simulink model "PMSM20180521"  (Simulink 7.9)
settings: Solver=FixedStepDiscrete  StartTime=0.0  StopTime=1  FixedStep=Auto  RelTol=1e-3
undefined symbols (not defined in the file or in its folder): Down, Up
libraries: idelinklib_common x37, simulink x13, c2833xlib x7, c280xlib x6, simulink_extras x2, idelinklib_ticcs x1, idelinklib_tgtpref x1
(part 2 of 3)

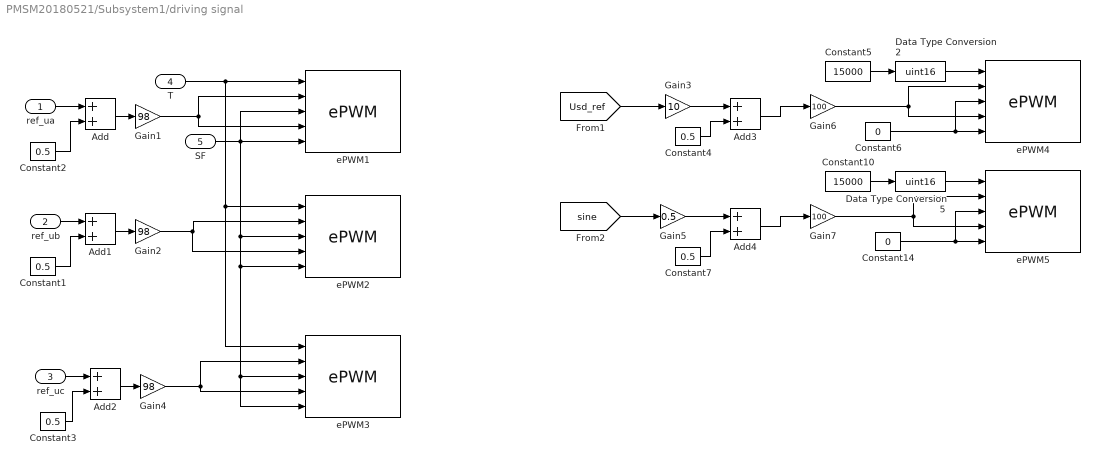
== system PMSM20180521/Subsystem1/driving signal ==
  ref_ua : Inport
  ref_ub : Inport  Port=2
  ref_uc : Inport  Port=3
  T : Inport  Port=4
  SF : Inport  Port=5
  Add{,1..4} (5 alike) : Sum
  Constant{1..4,7} (5 alike) : Constant  Value=0.5  OutDataTypeStr=double
  Constant10 : Constant  Value=15000  OutDataTypeStr=int16
  Constant14 : Constant  Value=0  OutDataTypeStr=boolean
  Constant5 : Constant  Value=15000  OutDataTypeStr=int16
  Constant6 : Constant  Value=0  OutDataTypeStr=boolean
  Data Type Conversion2 : DataTypeConversion  OutDataTypeStr=uint16
  Data Type Conversion5 : DataTypeConversion  OutDataTypeStr=uint16
  Gain1 : Gain  Gain=98
  Gain2 : Gain  Gain=98
  Gain3 : Gain  Gain=10
  Gain4 : Gain  Gain=98
  Gain5 : Gain  Gain=0.5
  Gain6 : Gain  Gain=100
  Gain7 : Gain  Gain=100
  ePWM1 : c280xlib/ePWM  checkMode=off  useModule=ePWM1  periodUnits=Clock cycles  timerSource=Input port  timerPeriod_clk=15000  timerPeriod_sec=1/20000  countingMode=Up-Down  synchronizationOption=CTR=Zero  synchronizationEnable=off  phaseActiveEnable=Disable  phaseDirection=Count down after sync  phaseActive=0  clockPrescale=1  HSclockPrescale=1  ePWMxAStatus=off  CMPAUnits=Percentages  CMPASource=Input port  CMPAValue_per=0  CMPAValue_clk=32000  ePWMxAactionLogic1=Do nothing  ePWMxAactionLogic2=Do nothing  ePWMxAactionLogic3=Clear  ePWMxAactionLogic4=Set  ePWMxAactionLogic5=Do nothing  ePWMxAactionLogic6=Do nothing  ePWMxALoadMode=Load on CTR=Zero  ePWMxACSFenable=on  ePWMxACSFvalue=Forcing Disable  ePWMxASFreload=Zero  enHRPWM=off  HRPWM_LoadMode=CTR=ZERO  HRPWM_CTLMode=Phase control mode  HRPWM_EDGMode=Both edge  enSFO=on  ePWMxBStatus=on  CMPBUnits=Percentages  CMPBSource=Input port  CMPBValue_per=0  CMPBValue_clk=32000  ePWMxBactionLogic1=Do nothing  ePWMxBactionLogic2=Do nothing  ePWMxBactionLogic3=Do nothing  ePWMxBactionLogic4=Do nothing  ePWMxBactionLogic5=Set  ePWMxBactionLogic6=Clear  ePWMxBLoadMode=Load on CTR=Zero  ePWMxBCSFenable=on  ePWMxBCSFvalue=Forcing Disable  ePWMxBSFreload=Zero  enableDBePWMxA=on  enableDBePWMxB=on  DBpolarity=AHC  DBedgeDelay=Positive  DBSource_ePWMxA=ePWMxB  DBSource_ePWMxB=ePWMxB  DBperiodSource=Specify via dialog  REDperiod=525  FEDperiod=525  adcstartModuleA=off  adcrequestEventA=First event  adcstartEventA=CTR=Zero  adcstartModuleB=off  adcrequestEventB=First event  adcstartEventB=CTR=Zero  intEn=on  intPrd=First event  intSel=CTR=Zero  chopperEnable=off  chopperFrequency=1  chopperFirstwidth=1  chopperDuty=12.5%  tripZonesource=Specify via dialog  tzselOSHT1=off  tzselOSHT2=off  tzselOSHT3=off  tzselOSHT4=off  tzselOSHT5=off  tzselOSHT6=off  tzselCBC1=off  tzselCBC2=off  tzselCBC3=off  tzselCBC4=off  tzselCBC5=off  tzselCBC6=off  enTzOstIntr=off  enTzCbcIntr=off  ePWMxAforced=No action  ePWMxBforced=No action  timerPeriod=-1  ePWMxAValue=0  ePWMxBValue=0  tripZoneoption=OSHT
  ePWM2 : c280xlib/ePWM  checkMode=off  useModule=ePWM2  periodUnits=Clock cycles  timerSource=Input port  timerPeriod_clk=15000  timerPeriod_sec=1/20000  countingMode=Up-Down  synchronizationOption=EPWMxSYNCI or SWFSYNC  synchronizationEnable=off  phaseActiveEnable=Specify via dialog  phaseDirection=Count up after sync  phaseActive=0  clockPrescale=1  HSclockPrescale=1  ePWMxAStatus=off  CMPAUnits=Percentages  CMPASource=Input port  CMPAValue_per=0  CMPAValue_clk=32000  ePWMxAactionLogic1=Do nothing  ePWMxAactionLogic2=Do nothing  ePWMxAactionLogic3=Clear  ePWMxAactionLogic4=Set  ePWMxAactionLogic5=Do nothing  ePWMxAactionLogic6=Do nothing  ePWMxALoadMode=Load on CTR=Zero  ePWMxACSFenable=on  ePWMxACSFvalue=Forcing Disable  ePWMxASFreload=Zero  enHRPWM=off  HRPWM_LoadMode=CTR=ZERO  HRPWM_CTLMode=Phase control mode  HRPWM_EDGMode=Both edge  enSFO=on  ePWMxBStatus=on  CMPBUnits=Percentages  CMPBSource=Input port  CMPBValue_per=0  CMPBValue_clk=32000  ePWMxBactionLogic1=Do nothing  ePWMxBactionLogic2=Do nothing  ePWMxBactionLogic3=Do nothing  ePWMxBactionLogic4=Do nothing  ePWMxBactionLogic5=Set  ePWMxBactionLogic6=Clear  ePWMxBLoadMode=Load on CTR=Zero  ePWMxBCSFenable=on  ePWMxBCSFvalue=Forcing Disable  ePWMxBSFreload=Zero  enableDBePWMxA=on  enableDBePWMxB=on  DBpolarity=AHC  DBedgeDelay=Positive  DBSource_ePWMxA=ePWMxB  DBSource_ePWMxB=ePWMxB  DBperiodSource=Specify via dialog  REDperiod=525  FEDperiod=525  adcstartModuleA=off  adcrequestEventA=First event  adcstartEventA=CTR=Zero  adcstartModuleB=off  adcrequestEventB=First event  adcstartEventB=CTR=Zero  intEn=off  intPrd=First event  intSel=CTR=Zero  chopperEnable=off  chopperFrequency=1  chopperFirstwidth=1  chopperDuty=12.5%  tripZonesource=Specify via dialog  tzselOSHT1=off  tzselOSHT2=off  tzselOSHT3=off  tzselOSHT4=off  tzselOSHT5=off  tzselOSHT6=off  tzselCBC1=off  tzselCBC2=off  tzselCBC3=off  tzselCBC4=off  tzselCBC5=off  tzselCBC6=off  enTzOstIntr=off  enTzCbcIntr=off  ePWMxAforced=No action  ePWMxBforced=No action  timerPeriod=-1  ePWMxAValue=0  ePWMxBValue=0  tripZoneoption=OSHT
  ePWM3 : c280xlib/ePWM  checkMode=off  useModule=ePWM3  periodUnits=Clock cycles  timerSource=Input port  timerPeriod_clk=15000  timerPeriod_sec=1/20000  countingMode=Up-Down  synchronizationOption=EPWMxSYNCI or SWFSYNC  synchronizationEnable=off  phaseActiveEnable=Specify via dialog  phaseDirection=Count up after sync  phaseActive=0  clockPrescale=1  HSclockPrescale=1  ePWMxAStatus=off  CMPAUnits=Percentages  CMPASource=Input port  CMPAValue_per=0  CMPAValue_clk=32000  ePWMxAactionLogic1=Do nothing  ePWMxAactionLogic2=Do nothing  ePWMxAactionLogic3=Clear  ePWMxAactionLogic4=Set  ePWMxAactionLogic5=Do nothing  ePWMxAactionLogic6=Do nothing  ePWMxALoadMode=Load on CTR=Zero  ePWMxACSFenable=on  ePWMxACSFvalue=Forcing Disable  ePWMxASFreload=Zero  enHRPWM=off  HRPWM_LoadMode=CTR=ZERO  HRPWM_CTLMode=Phase control mode  HRPWM_EDGMode=Both edge  enSFO=on  ePWMxBStatus=on  CMPBUnits=Percentages  CMPBSource=Input port  CMPBValue_per=0  CMPBValue_clk=32000  ePWMxBactionLogic1=Do nothing  ePWMxBactionLogic2=Do nothing  ePWMxBactionLogic3=Do nothing  ePWMxBactionLogic4=Do nothing  ePWMxBactionLogic5=Set  ePWMxBactionLogic6=Clear  ePWMxBLoadMode=Load on CTR=Zero  ePWMxBCSFenable=on  ePWMxBCSFvalue=Forcing Disable  ePWMxBSFreload=Zero  enableDBePWMxA=on  enableDBePWMxB=on  DBpolarity=AHC  DBedgeDelay=Positive  DBSource_ePWMxA=ePWMxB  DBSource_ePWMxB=ePWMxB  DBperiodSource=Specify via dialog  REDperiod=525  FEDperiod=525  adcstartModuleA=off  adcrequestEventA=First event  adcstartEventA=CTR=Zero  adcstartModuleB=off  adcrequestEventB=First event  adcstartEventB=CTR=Zero  intEn=off  intPrd=First event  intSel=CTR=Zero  chopperEnable=off  chopperFrequency=1  chopperFirstwidth=1  chopperDuty=12.5%  tripZonesource=Specify via dialog  tzselOSHT1=off  tzselOSHT2=off  tzselOSHT3=off  tzselOSHT4=off  tzselOSHT5=off  tzselOSHT6=off  tzselCBC1=off  tzselCBC2=off  tzselCBC3=off  tzselCBC4=off  tzselCBC5=off  tzselCBC6=off  enTzOstIntr=off  enTzCbcIntr=off  ePWMxAforced=No action  ePWMxBforced=No action  timerPeriod=-1  ePWMxAValue=0  ePWMxBValue=0  tripZoneoption=OSHT
  ePWM4 : c280xlib/ePWM  checkMode=off  useModule=ePWM4  periodUnits=Clock cycles  timerSource=Input port  timerPeriod_clk=15000  timerPeriod_sec=1/20000  countingMode=Up-Down  synchronizationOption=EPWMxSYNCI or SWFSYNC  synchronizationEnable=off  phaseActiveEnable=Specify via dialog  phaseDirection=Count up after sync  phaseActive=0  clockPrescale=1  HSclockPrescale=1  ePWMxAStatus=on  CMPAUnits=Percentages  CMPASource=Input port  CMPAValue_per=0  CMPAValue_clk=32000  ePWMxAactionLogic1=Do nothing  ePWMxAactionLogic2=Do nothing  ePWMxAactionLogic3=Clear  ePWMxAactionLogic4=Set  ePWMxAactionLogic5=Do nothing  ePWMxAactionLogic6=Do nothing  ePWMxALoadMode=Load on CTR=Zero  ePWMxACSFenable=on  ePWMxACSFvalue=Forcing Disable  ePWMxASFreload=Zero  enHRPWM=off  HRPWM_LoadMode=CTR=ZERO  HRPWM_CTLMode=Phase control mode  HRPWM_EDGMode=Both edge  enSFO=on  ePWMxBStatus=on  CMPBUnits=Percentages  CMPBSource=Input port  CMPBValue_per=0  CMPBValue_clk=32000  ePWMxBactionLogic1=Do nothing  ePWMxBactionLogic2=Do nothing  ePWMxBactionLogic3=Do nothing  ePWMxBactionLogic4=Do nothing  ePWMxBactionLogic5=Clear  ePWMxBactionLogic6=Set  ePWMxBLoadMode=Load on CTR=Zero  ePWMxBCSFenable=on  ePWMxBCSFvalue=Forcing Disable  ePWMxBSFreload=Zero  enableDBePWMxA=off  enableDBePWMxB=off  DBpolarity=AHC  DBedgeDelay=Positive  DBSource_ePWMxA=ePWMxB  DBSource_ePWMxB=ePWMxB  DBperiodSource=Specify via dialog  REDperiod=0  FEDperiod=0  adcstartModuleA=off  adcrequestEventA=First event  adcstartEventA=CTR=Zero  adcstartModuleB=off  adcrequestEventB=First event  adcstartEventB=CTR=Zero  intEn=off  intPrd=First event  intSel=CTR=Zero  chopperEnable=off  chopperFrequency=1  chopperFirstwidth=1  chopperDuty=12.5%  tripZonesource=Specify via dialog  tzselOSHT1=off  tzselOSHT2=off  tzselOSHT3=off  tzselOSHT4=off  tzselOSHT5=off  tzselOSHT6=off  tzselCBC1=off  tzselCBC2=off  tzselCBC3=off  tzselCBC4=off  tzselCBC5=off  tzselCBC6=off  enTzOstIntr=off  enTzCbcIntr=off  ePWMxAforced=No action  ePWMxBforced=No action  timerPeriod=-1  ePWMxAValue=0  ePWMxBValue=0  tripZoneoption=OSHT
  ePWM5 : c280xlib/ePWM  checkMode=off  useModule=ePWM5  periodUnits=Clock cycles  timerSource=Input port  timerPeriod_clk=15000  timerPeriod_sec=1/20000  countingMode=Up-Down  synchronizationOption=EPWMxSYNCI or SWFSYNC  synchronizationEnable=off  phaseActiveEnable=Specify via dialog  phaseDirection=Count up after sync  phaseActive=0  clockPrescale=1  HSclockPrescale=1  ePWMxAStatus=on  CMPAUnits=Percentages  CMPASource=Input port  CMPAValue_per=0  CMPAValue_clk=32000  ePWMxAactionLogic1=Do nothing  ePWMxAactionLogic2=Do nothing  ePWMxAactionLogic3=Clear  ePWMxAactionLogic4=Set  ePWMxAactionLogic5=Do nothing  ePWMxAactionLogic6=Do nothing  ePWMxALoadMode=Load on CTR=Zero  ePWMxACSFenable=on  ePWMxACSFvalue=Forcing Disable  ePWMxASFreload=Zero  enHRPWM=off  HRPWM_LoadMode=CTR=ZERO  HRPWM_CTLMode=Phase control mode  HRPWM_EDGMode=Both edge  enSFO=on  ePWMxBStatus=on  CMPBUnits=Percentages  CMPBSource=Input port  CMPBValue_per=0  CMPBValue_clk=32000  ePWMxBactionLogic1=Do nothing  ePWMxBactionLogic2=Do nothing  ePWMxBactionLogic3=Do nothing  ePWMxBactionLogic4=Do nothing  ePWMxBactionLogic5=Clear  ePWMxBactionLogic6=Set  ePWMxBLoadMode=Load on CTR=Zero  ePWMxBCSFenable=on  ePWMxBCSFvalue=Forcing Disable  ePWMxBSFreload=Zero  enableDBePWMxA=off  enableDBePWMxB=off  DBpolarity=AHC  DBedgeDelay=Positive  DBSource_ePWMxA=ePWMxB  DBSource_ePWMxB=ePWMxB  DBperiodSource=Specify via dialog  REDperiod=0  FEDperiod=0  adcstartModuleA=off  adcrequestEventA=First event  adcstartEventA=CTR=Zero  adcstartModuleB=off  adcrequestEventB=First event  adcstartEventB=CTR=Zero  intEn=off  intPrd=First event  intSel=CTR=Zero  chopperEnable=off  chopperFrequency=1  chopperFirstwidth=1  chopperDuty=12.5%  tripZonesource=Specify via dialog  tzselOSHT1=off  tzselOSHT2=off  tzselOSHT3=off  tzselOSHT4=off  tzselOSHT5=off  tzselOSHT6=off  tzselCBC1=off  tzselCBC2=off  tzselCBC3=off  tzselCBC4=off  tzselCBC5=off  tzselCBC6=off  enTzOstIntr=off  enTzCbcIntr=off  ePWMxAforced=No action  ePWMxBforced=No action  timerPeriod=-1  ePWMxAValue=0  ePWMxBValue=0  tripZoneoption=OSHT
  wires:
  SF/1 -> ePWM1/3, ePWM1/5, ePWM3/5, ePWM3/3, ePWM2/5, ePWM2/3
  T/1 -> ePWM1/1, ePWM3/1, ePWM2/1
  ref_ua/1 -> Add/1
  Add/1 -> Gain1/1
  Constant2/1 -> Add/2
  Gain1/1 -> ePWM1/2, ePWM1/4
  ref_ub/1 -> Add1/1
  Constant1/1 -> Add1/2
  Add1/1 -> Gain2/1
  Gain2/1 -> ePWM2/4, ePWM2/2
  ref_uc/1 -> Add2/1
  Constant3/1 -> Add2/2
  Add2/1 -> Gain4/1
  Gain4/1 -> ePWM3/2, ePWM3/4
  Data Type Conversion5/1 -> ePWM5/1
  Constant14/1 -> ePWM5/3, ePWM5/5
  Constant5/1 -> Data Type Conversion2/1
  Gain7/1 -> ePWM5/2, ePWM5/4
  Data Type Conversion2/1 -> ePWM4/1
  Gain6/1 -> ePWM4/4, ePWM4/2
  Constant10/1 -> Data Type Conversion5/1
  Constant6/1 -> ePWM4/3, ePWM4/5
  [sine] -> Gain5/1
  [Usd_ref] -> Gain3/1
  Gain3/1 -> Add3/1
  Add3/1 -> Gain6/1
  Constant4/1 -> Add3/2
  Gain5/1 -> Add4/1
  Add4/1 -> Gain7/1
  Constant7/1 -> Add4/2

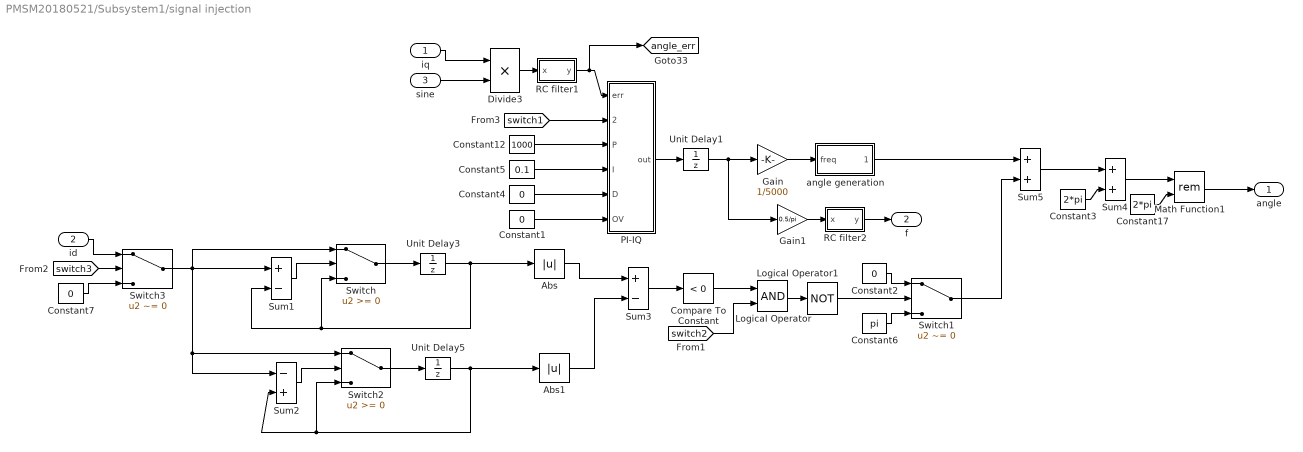
== system PMSM20180521/Subsystem1/signal injection ==
  iq : Inport
  id : Inport  Port=2
  sine : Inport  Port=3
  Abs : Abs
  Abs1 : Abs
  Compare To Constant : simulink/Logic and Bit Operations/Compare To Constant  relop=<  const=0  OutDataTypeStr=boolean
  Constant{1..2,4,7} (4 alike) : Constant  Value=0  OutDataTypeStr=double
  Constant12 : Constant  Value=1000  OutDataTypeStr=double
  Constant17 : Constant  Value=2*pi  OutDataTypeStr=double
  Constant3 : Constant  Value=2*pi  OutDataTypeStr=double
  Constant5 : Constant  Value=0.1  OutDataTypeStr=double
  Constant6 : Constant  Value=pi  OutDataTypeStr=double
  Divide3 : Product  Inputs=**
  Gain : Gain  Gain=1/5000
  Gain1 : Gain  Gain=0.5/pi
  Logical Operator : Logic  AllPortsSameDT=off  OutDataTypeStr=boolean
  Logical Operator1 : Logic  Operator=NOT  AllPortsSameDT=off  OutDataTypeStr=boolean
  Math Function1 : Math  Operator=rem  SaturateOnIntegerOverflow=on
  PI-IQ : Subsystem  mask{ermax=100, ermin=-100, max=300, min=-300}
      mask prompts: ermax "Err max limit"; ermin "Err min limit"; max "Output max limit"; min "Output min limit"
  RC filter1 : Subsystem  mask{a=0.05}
      mask prompts: a "Time Constant"
  RC filter2 : Subsystem  mask{a=0.05}
      mask prompts: a "Time Constant"
  Sum1 : Sum  Inputs=+-
  Sum2 : Sum  Inputs=-+
  Sum3 : Sum  Inputs=+-
  Sum4 : Sum
  Sum5 : Sum
  Switch : Switch
  Switch1 : Switch  Criteria=u2 ~= 0
  Switch2 : Switch
  Switch3 : Switch  Criteria=u2 ~= 0
  Unit Delay1 : UnitDelay  SampleTime=-1
  Unit Delay3 : UnitDelay  SampleTime=-1
  Unit Delay5 : UnitDelay  SampleTime=-1
  angle generation : Subsystem
  angle : Outport
  f : Outport  Port=2
  tag scope: angle_err=global
  wires:
  sine/1 -> Divide3/2
  Divide3/1 -> RC filter1/1(x)
  Constant12/1 -> PI-IQ/3(P)
  Constant5/1 -> PI-IQ/4(I)
  Constant4/1 -> PI-IQ/5(D)
  Constant1/1 -> PI-IQ/6(OV)
  RC filter1/1(y) -> PI-IQ/1(err), [angle_err]
  PI-IQ/1(out) -> Unit Delay1/1
  iq/1 -> Divide3/1
  Gain/1 -> angle generation/1(freq)
  Unit Delay1/1 -> Gain/1, Gain1/1
  Gain1/1 -> RC filter2/1(x)
  Constant3/1 -> Sum4/2
  Constant17/1 -> Math Function1/2
  Sum4/1 -> Math Function1/1
  Math Function1/1 -> angle/1
  RC filter2/1(y) -> f/1
  [switch1] -> PI-IQ/2(reset)
  Sum1/1 -> Switch/2
  Switch/1 -> Unit Delay3/1
  Unit Delay3/1 -> Sum1/2, Switch/3, Abs/1
  Sum2/1 -> Switch2/2
  Switch2/1 -> Unit Delay5/1
  Unit Delay5/1 -> Sum2/2, Switch2/3, Abs1/1
  Abs/1 -> Sum3/1
  Abs1/1 -> Sum3/2
  Constant2/1 -> Switch1/1
  Constant6/1 -> Switch1/3
  Sum3/1 -> Compare To Constant/1
  Compare To Constant/1 -> Logical Operator/1
  [switch2] -> Logical Operator/2
  Logical Operator/1 -> Logical Operator1/1
  Logical Operator1/1 -> Switch1/2
  Switch3/1 -> Sum1/1, Switch/1, Sum2/1, Switch2/1
  [switch3] -> Switch3/2
  id/1 -> Switch3/1
  Constant7/1 -> Switch3/3
  Sum5/1 -> Sum4/1
  Switch1/1 -> Sum5/2
  angle generation/1(angle_0) -> Sum5/1

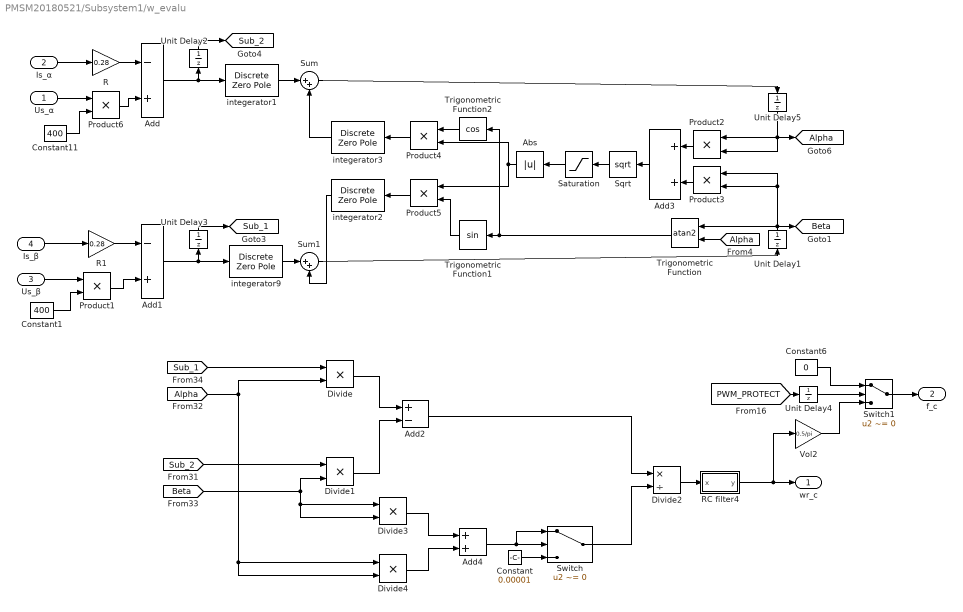
== system PMSM20180521/Subsystem1/w_evalu ==
  Us_α : Inport
  Is_α : Inport  Port=2
  Us_β : Inport  Port=3
  Is_β : Inport  Port=4
  Abs : Abs
  Add : Sum  Inputs=-+
  Add1 : Sum  Inputs=-+
  Add2 : Sum  Inputs=+-
  Add3 : Sum
  Add4 : Sum
  Constant : Constant  Value=0.00001
  Constant1 : Constant  Value=400  OutDataTypeStr=double
  Constant11 : Constant  Value=400  OutDataTypeStr=double
  Constant6 : Constant  Value=0  OutDataTypeStr=double
  Divide{,1,3..4} (4 alike) : Product  Inputs=**
  Divide2 : Product  Inputs=*/
  Product{1..6} (6 alike) : Product  RndMeth=Zero
  R : Gain  Gain=0.28
  R1 : Gain  Gain=0.28
  RC filter4 : Subsystem  mask{a=0.2}
      mask prompts: a "Time Constant"
  Saturation : Saturate  UpperLimit=0.56  LowerLimit=-0.56
  Sqrt : Sqrt  SaturateOnIntegerOverflow=on
  Sum : Sum  Inputs=|++
  Sum1 : Sum  Inputs=|++
  Switch : Switch  Criteria=u2 ~= 0
  Switch1 : Switch  Criteria=u2 ~= 0
  Trigonometric Function : Trigonometry  Operator=atan2
  Trigonometric Function1 : Trigonometry
  Trigonometric Function2 : Trigonometry  Operator=cos
  Unit Delay{1..5} (5 alike) : UnitDelay  SampleTime=-1
  Vol2 : Gain  Gain=0.5/pi
  integerator1 : DiscreteZeroPole  Zeros=[0]  Poles=[1/1.03]  Gain=0.0002/1.03  SampleTime=-1
  integerator2 : DiscreteZeroPole  Zeros=[0]  Poles=[1/1.03]  Gain=0.0002/1.03*150  SampleTime=-1
  integerator3 : DiscreteZeroPole  Zeros=[0]  Poles=[1/1.03]  Gain=0.0002/1.03*150  SampleTime=-1
  integerator9 : DiscreteZeroPole  Zeros=[0]  Poles=[1/1.03]  Gain=0.0002/1.03  SampleTime=-1
  wr_c : Outport
  f_c : Outport  Port=2
  tag scope: Alpha=global, Beta=global, Sub_1=global, Sub_2=global
  wires:
  Product6/1 -> Add/2
  Add/1 -> Unit Delay2/1, integerator1/1
  Us_α/1 -> Product6/1
  Is_α/1 -> R/1
  R/1 -> Add/1
  R1/1 -> Add1/1
  Is_β/1 -> R1/1
  Us_β/1 -> Product1/1
  Add1/1 -> integerator9/1, Unit Delay3/1
  Product1/1 -> Add1/2
  integerator1/1 -> Sum/1
  integerator9/1 -> Sum1/1
  Sum/1 -> Unit Delay5/1
  Sum1/1 -> Unit Delay1/1
  Product3/1 -> Add3/2
  Product2/1 -> Add3/1
  Add3/1 -> Sqrt/1
  Product4/1 -> integerator3/1
  Product5/1 -> integerator2/1
  Abs/1 -> Product4/2, Product5/1
  Unit Delay1/1 -> [Beta], Product3/1, Product3/2, Trigonometric Function/1
  Unit Delay5/1 -> Product2/2, Product2/1, [Alpha]
  Unit Delay2/1 -> [Sub_2]
  Unit Delay3/1 -> [Sub_1]
  Sqrt/1 -> Saturation/1
  Saturation/1 -> Abs/1
  [Alpha] -> Trigonometric Function/2
  Trigonometric Function/1 -> Trigonometric Function1/1, Trigonometric Function2/1
  Trigonometric Function1/1 -> Product5/2
  Trigonometric Function2/1 -> Product4/1
  integerator2/1 -> Sum1/2
  integerator3/1 -> Sum/2
  [Sub_1] -> Divide/1
  [Alpha] -> Divide/2, Divide4/1, Divide4/2
  [Sub_2] -> Divide1/1
  [Beta] -> Divide1/2, Divide3/1, Divide3/2
  Divide/1 -> Add2/1
  Divide1/1 -> Add2/2
  Add2/1 -> Divide2/1
  Divide3/1 -> Add4/1
  Divide4/1 -> Add4/2
  Divide2/1 -> RC filter4/1(x)
  Add4/1 -> Switch/2, Switch/1
  Switch/1 -> Divide2/2
  Constant/1 -> Switch/3
  RC filter4/1(y) -> wr_c/1, Vol2/1
  Switch1/1 -> f_c/1
  [PWM_PROTECT] -> Unit Delay4/1
  Constant6/1 -> Switch1/1
  Unit Delay4/1 -> Switch1/2
  Vol2/1 -> Switch1/3
  Constant1/1 -> Product1/2
  Constant11/1 -> Product6/2

== system PMSM20180521/Function-Call Subsystem1/Subsystem1/求个位 ==
  In1 : Inport
  In2 : Inport  Port=2
  In3 : Inport  Port=3
  Constant1 : Constant  OutDataTypeStr=uint16
  Gain : Gain  Gain=100
  Gain1 : Gain  Gain=10
  Math Function : Math  Operator=rem  SaturateOnIntegerOverflow=on
  Product : Product  Inputs=*/
  Sum : Sum  Inputs=+--  AccumDataTypeStr=uint16  OutDataTypeStr=uint16
  Sum1 : Sum  Inputs=+-
  Out1 : Outport
  wires:
  In2/1 -> Gain/1
  In3/1 -> Gain1/1
  In1/1 -> Sum/1
  Gain/1 -> Sum/2
  Gain1/1 -> Sum/3
  Sum1/1 -> Product/1
  Math Function/1 -> Sum1/2
  Constant1/1 -> Math Function/2, Product/2
  Product/1 -> Out1/1
  Sum/1 -> Math Function/1, Sum1/1

== system PMSM20180521/Function-Call Subsystem1/Subsystem1/求十位 ==
  In1 : Inport
  In2 : Inport  Port=2
  Constant1 : Constant  Value=10  OutDataTypeStr=uint16
  Gain1 : Gain  Gain=100
  Math Function : Math  Operator=rem  SaturateOnIntegerOverflow=on
  Product : Product  Inputs=*/
  Sum : Sum  Inputs=+-
  Sum1 : Sum  Inputs=+-  OutDataTypeStr=uint16
  Out1 : Outport
  wires:
  Sum/1 -> Product/1
  Math Function/1 -> Sum/2
  Constant1/1 -> Math Function/2, Product/2
  Product/1 -> Out1/1
  In1/1 -> Gain1/1
  In2/1 -> Sum1/1
  Gain1/1 -> Sum1/2
  Sum1/1 -> Sum/1, Math Function/1

== system PMSM20180521/Function-Call Subsystem1/Subsystem1/求百位 ==
  In1 : Inport
  Constant1 : Constant  Value=100  OutDataTypeStr=uint16
  Math Function : Math  Operator=rem  SaturateOnIntegerOverflow=on
  Product : Product  Inputs=*/
  Sum : Sum  Inputs=+-
  Out1 : Outport
  wires:
  Product/1 -> Out1/1
  Constant1/1 -> Product/2, Math Function/2
  In1/1 -> Sum/1, Math Function/1
  Math Function/1 -> Sum/2
  Sum/1 -> Product/1

== system PMSM20180521/Function-Call Subsystem1/Subsystem2/求个位 ==
  In1 : Inport
  In2 : Inport  Port=2
  In3 : Inport  Port=3
  Constant1 : Constant  OutDataTypeStr=uint16
  Gain : Gain  Gain=100
  Gain1 : Gain  Gain=10
  Math Function : Math  Operator=rem  SaturateOnIntegerOverflow=on
  Product : Product  Inputs=*/
  Sum : Sum  Inputs=+--  AccumDataTypeStr=uint16  OutDataTypeStr=uint16
  Sum1 : Sum  Inputs=+-
  Out1 : Outport
  wires:
  Sum/1 -> Sum1/1, Math Function/1
  Product/1 -> Out1/1
  Constant1/1 -> Product/2, Math Function/2
  Math Function/1 -> Sum1/2
  Sum1/1 -> Product/1
  Gain1/1 -> Sum/3
  Gain/1 -> Sum/2
  In1/1 -> Sum/1
  In3/1 -> Gain1/1
  In2/1 -> Gain/1

== system PMSM20180521/Function-Call Subsystem1/Subsystem2/求十位 ==
  In1 : Inport
  In2 : Inport  Port=2
  Constant1 : Constant  Value=10  OutDataTypeStr=uint16
  Gain1 : Gain  Gain=100
  Math Function : Math  Operator=rem  SaturateOnIntegerOverflow=on
  Product : Product  Inputs=*/
  Sum : Sum  Inputs=+-
  Sum1 : Sum  Inputs=+-  OutDataTypeStr=uint16
  Out1 : Outport
  wires:
  Sum1/1 -> Math Function/1, Sum/1
  Gain1/1 -> Sum1/2
  In2/1 -> Sum1/1
  In1/1 -> Gain1/1
  Product/1 -> Out1/1
  Constant1/1 -> Product/2, Math Function/2
  Math Function/1 -> Sum/2
  Sum/1 -> Product/1

== system PMSM20180521/Function-Call Subsystem1/Subsystem2/求百位 ==
  In1 : Inport
  Constant1 : Constant  Value=100  OutDataTypeStr=uint16
  Math Function : Math  Operator=rem  SaturateOnIntegerOverflow=on
  Product : Product  Inputs=*/
  Sum : Sum  Inputs=+-
  Out1 : Outport
  wires:
  Sum/1 -> Product/1
  Math Function/1 -> Sum/2
  In1/1 -> Math Function/1, Sum/1
  Constant1/1 -> Math Function/2, Product/2
  Product/1 -> Out1/1

== system PMSM20180521/Function-Call Subsystem1/Subsystem3/求个位 ==
  In1 : Inport
  In2 : Inport  Port=2
  In3 : Inport  Port=3
  Constant1 : Constant  OutDataTypeStr=uint16
  Gain : Gain  Gain=100
  Gain1 : Gain  Gain=10
  Math Function : Math  Operator=rem  SaturateOnIntegerOverflow=on
  Product : Product  Inputs=*/
  Sum : Sum  Inputs=+--  AccumDataTypeStr=uint16  OutDataTypeStr=uint16
  Sum1 : Sum  Inputs=+-
  Out1 : Outport
  wires:
  In2/1 -> Gain/1
  In3/1 -> Gain1/1
  In1/1 -> Sum/1
  Gain/1 -> Sum/2
  Gain1/1 -> Sum/3
  Sum1/1 -> Product/1
  Math Function/1 -> Sum1/2
  Constant1/1 -> Math Function/2, Product/2
  Product/1 -> Out1/1
  Sum/1 -> Math Function/1, Sum1/1

== system PMSM20180521/Function-Call Subsystem1/Subsystem3/求十位 ==
  In1 : Inport
  In2 : Inport  Port=2
  Constant1 : Constant  Value=10  OutDataTypeStr=uint16
  Gain1 : Gain  Gain=100
  Math Function : Math  Operator=rem  SaturateOnIntegerOverflow=on
  Product : Product  Inputs=*/
  Sum : Sum  Inputs=+-
  Sum1 : Sum  Inputs=+-  OutDataTypeStr=uint16
  Out1 : Outport
  wires:
  Sum/1 -> Product/1
  Math Function/1 -> Sum/2
  Constant1/1 -> Math Function/2, Product/2
  Product/1 -> Out1/1
  In1/1 -> Gain1/1
  In2/1 -> Sum1/1
  Gain1/1 -> Sum1/2
  Sum1/1 -> Sum/1, Math Function/1

== system PMSM20180521/Function-Call Subsystem1/Subsystem3/求百位 ==
  In1 : Inport
  Constant1 : Constant  Value=100  OutDataTypeStr=uint16
  Math Function : Math  Operator=rem  SaturateOnIntegerOverflow=on
  Product : Product  Inputs=*/
  Sum : Sum  Inputs=+-
  Out1 : Outport
  wires:
  Product/1 -> Out1/1
  Constant1/1 -> Product/2, Math Function/2
  In1/1 -> Sum/1, Math Function/1
  Math Function/1 -> Sum/2
  Sum/1 -> Product/1

== system PMSM20180521/Subsystem1/AD/Start Conversion ==
  Constant : Constant  Value=0  OutDataTypeStr=boolean
  Digital Output1 : c2833xlib/Digital Output  Priority=1  GPIO_Number=GPIO48~GPIO55  GPIO_Bit0=off  GPIO_BIT0_Toggle=off  GPIO_Bit1=on  GPIO_BIT1_Toggle=off  GPIO_Bit2=off  GPIO_BIT2_Toggle=off  GPIO_Bit3=off  GPIO_BIT3_Toggle=off  GPIO_Bit4=off  GPIO_BIT4_Toggle=off  GPIO_Bit5=off  GPIO_BIT5_Toggle=off  GPIO_Bit6=off  GPIO_BIT6_Toggle=off  GPIO_Bit7=off  GPIO_BIT7_Toggle=off
  wires:
  Constant/1 -> Digital Output1/1

== system PMSM20180521/Subsystem1/AD/Stop Conversion ==
  Constant12 : Constant  OutDataTypeStr=boolean
  Digital Output13 : c2833xlib/Digital Output  Priority=8  GPIO_Number=GPIO48~GPIO55  GPIO_Bit0=off  GPIO_BIT0_Toggle=off  GPIO_Bit1=on  GPIO_BIT1_Toggle=off  GPIO_Bit2=off  GPIO_BIT2_Toggle=off  GPIO_Bit3=off  GPIO_BIT3_Toggle=off  GPIO_Bit4=off  GPIO_BIT4_Toggle=off  GPIO_Bit5=off  GPIO_BIT5_Toggle=off  GPIO_Bit6=off  GPIO_BIT6_Toggle=off  GPIO_Bit7=off  GPIO_BIT7_Toggle=off
  wires:
  Constant12/1 -> Digital Output13/1

== system PMSM20180521/Subsystem1/AD/read AD ==
  CH0 : idelinklib_common/Memory Copy  copyFrom=Specified address  copyFromAddressSource=Specify via dialog  copyFromAddress=hex2dec('00200000')  copyFromSrcCode=myVariableSrc  dataTypeFrom=int16  dataDimensionFrom=1  useOffsetFrom=off  offsetFromSrc=Specify via dialog  offsetFrom=0  strideFrom=1  copyTo=Specified source code symbol  copyToAddressSource=Specify via dialog  copyToAddress=hex2dec('00002000')  copyToSrcCode=p1  dataTypeTo=int16  useOffsetTo=off  offsetToSrc=Specify via dialog  offsetTo=0  strideTo=1  sampleTime=inf  useInitValue=off  initValueSrc=Specify constant value  initValue=1  initValueSrcCode=myInitValueVariable  useAsMask=off  maskOperator=bitwise AND  useTermValue=off  termValue=1  isRealtimeEnabled=off  emitCCBeforeWrite=off  CCBeforeWrite=/* Custom Code Before Write*/  emitCCAfterWrite=off  CCAfterWrite=/* Custom Code After Write*/  useDMACopy=off  enableBlockingMode=off
  CH1 : idelinklib_common/Memory Copy  copyFrom=Specified address  copyFromAddressSource=Specify via dialog  copyFromAddress=hex2dec('00200000')  copyFromSrcCode=myVariableSrc  dataTypeFrom=int16  dataDimensionFrom=1  useOffsetFrom=off  offsetFromSrc=Specify via dialog  offsetFrom=0  strideFrom=1  copyTo=Specified source code symbol  copyToAddressSource=Specify via dialog  copyToAddress=hex2dec('00002000')  copyToSrcCode=p2  dataTypeTo=int16  useOffsetTo=off  offsetToSrc=Specify via dialog  offsetTo=0  strideTo=1  sampleTime=inf  useInitValue=off  initValueSrc=Specify constant value  initValue=1  initValueSrcCode=myInitValueVariable  useAsMask=off  maskOperator=bitwise AND  useTermValue=off  termValue=1  isRealtimeEnabled=off  emitCCBeforeWrite=off  CCBeforeWrite=/* Custom Code Before Write*/  emitCCAfterWrite=off  CCAfterWrite=/* Custom Code After Write*/  useDMACopy=off  enableBlockingMode=off
  CH2 : idelinklib_common/Memory Copy  copyFrom=Specified address  copyFromAddressSource=Specify via dialog  copyFromAddress=hex2dec('00200000')  copyFromSrcCode=myVariableSrc  dataTypeFrom=int16  dataDimensionFrom=1  useOffsetFrom=off  offsetFromSrc=Specify via dialog  offsetFrom=0  strideFrom=1  copyTo=Specified source code symbol  copyToAddressSource=Specify via dialog  copyToAddress=hex2dec('00002000')  copyToSrcCode=p3  dataTypeTo=int16  useOffsetTo=off  offsetToSrc=Specify via dialog  offsetTo=0  strideTo=1  sampleTime=inf  useInitValue=off  initValueSrc=Specify constant value  initValue=1  initValueSrcCode=myInitValueVariable  useAsMask=off  maskOperator=bitwise AND  useTermValue=off  termValue=1  isRealtimeEnabled=off  emitCCBeforeWrite=off  CCBeforeWrite=/* Custom Code Before Write*/  emitCCAfterWrite=off  CCAfterWrite=/* Custom Code After Write*/  useDMACopy=off  enableBlockingMode=off
  CH3 : idelinklib_common/Memory Copy  copyFrom=Specified address  copyFromAddressSource=Specify via dialog  copyFromAddress=hex2dec('00200000')  copyFromSrcCode=myVariableSrc  dataTypeFrom=int16  dataDimensionFrom=1  useOffsetFrom=off  offsetFromSrc=Specify via dialog  offsetFrom=0  strideFrom=1  copyTo=Specified source code symbol  copyToAddressSource=Specify via dialog  copyToAddress=hex2dec('00002000')  copyToSrcCode=p4  dataTypeTo=int16  useOffsetTo=off  offsetToSrc=Specify via dialog  offsetTo=0  strideTo=1  sampleTime=inf  useInitValue=off  initValueSrc=Specify constant value  initValue=1  initValueSrcCode=myInitValueVariable  useAsMask=off  maskOperator=bitwise AND  useTermValue=off  termValue=1  isRealtimeEnabled=off  emitCCBeforeWrite=off  CCBeforeWrite=/* Custom Code Before Write*/  emitCCAfterWrite=off  CCAfterWrite=/* Custom Code After Write*/  useDMACopy=off  enableBlockingMode=off
  CH4 : idelinklib_common/Memory Copy  copyFrom=Specified address  copyFromAddressSource=Specify via dialog  copyFromAddress=hex2dec('00200000')  copyFromSrcCode=myVariableSrc  dataTypeFrom=int16  dataDimensionFrom=1  useOffsetFrom=off  offsetFromSrc=Specify via dialog  offsetFrom=0  strideFrom=1  copyTo=Specified source code symbol  copyToAddressSource=Specify via dialog  copyToAddress=hex2dec('00002000')  copyToSrcCode=p5  dataTypeTo=int16  useOffsetTo=off  offsetToSrc=Specify via dialog  offsetTo=0  strideTo=1  sampleTime=inf  useInitValue=off  initValueSrc=Specify constant value  initValue=1  initValueSrcCode=myInitValueVariable  useAsMask=off  maskOperator=bitwise AND  useTermValue=off  termValue=1  isRealtimeEnabled=off  emitCCBeforeWrite=off  CCBeforeWrite=/* Custom Code Before Write*/  emitCCAfterWrite=off  CCAfterWrite=/* Custom Code After Write*/  useDMACopy=off  enableBlockingMode=off
  CH5 : idelinklib_common/Memory Copy  copyFrom=Specified address  copyFromAddressSource=Specify via dialog  copyFromAddress=hex2dec('00200000')  copyFromSrcCode=myVariableSrc  dataTypeFrom=int16  dataDimensionFrom=1  useOffsetFrom=off  offsetFromSrc=Specify via dialog  offsetFrom=0  strideFrom=1  copyTo=Specified source code symbol  copyToAddressSource=Specify via dialog  copyToAddress=hex2dec('00002000')  copyToSrcCode=p6  dataTypeTo=int16  useOffsetTo=off  offsetToSrc=Specify via dialog  offsetTo=0  strideTo=1  sampleTime=inf  useInitValue=off  initValueSrc=Specify constant value  initValue=1  initValueSrcCode=myInitValueVariable  useAsMask=off  maskOperator=bitwise AND  useTermValue=off  termValue=1  isRealtimeEnabled=off  emitCCBeforeWrite=off  CCBeforeWrite=/* Custom Code Before Write*/  emitCCAfterWrite=off  CCAfterWrite=/* Custom Code After Write*/  useDMACopy=off  enableBlockingMode=off
  CH6 : idelinklib_common/Memory Copy  copyFrom=Specified address  copyFromAddressSource=Specify via dialog  copyFromAddress=hex2dec('00200000')  copyFromSrcCode=myVariableSrc  dataTypeFrom=int16  dataDimensionFrom=1  useOffsetFrom=off  offsetFromSrc=Specify via dialog  offsetFrom=0  strideFrom=1  copyTo=Specified source code symbol  copyToAddressSource=Specify via dialog  copyToAddress=hex2dec('00002000')  copyToSrcCode=p7  dataTypeTo=int16  useOffsetTo=off  offsetToSrc=Specify via dialog  offsetTo=0  strideTo=1  sampleTime=inf  useInitValue=off  initValueSrc=Specify constant value  initValue=1  initValueSrcCode=myInitValueVariable  useAsMask=off  maskOperator=bitwise AND  useTermValue=off  termValue=1  isRealtimeEnabled=off  emitCCBeforeWrite=off  CCBeforeWrite=/* Custom Code Before Write*/  emitCCAfterWrite=off  CCAfterWrite=/* Custom Code After Write*/  useDMACopy=off  enableBlockingMode=off
  CH7 : idelinklib_common/Memory Copy  copyFrom=Specified address  copyFromAddressSource=Specify via dialog  copyFromAddress=hex2dec('00200000')  copyFromSrcCode=myVariableSrc  dataTypeFrom=int16  dataDimensionFrom=1  useOffsetFrom=off  offsetFromSrc=Specify via dialog  offsetFrom=0  strideFrom=1  copyTo=Specified source code symbol  copyToAddressSource=Specify via dialog  copyToAddress=hex2dec('00002000')  copyToSrcCode=p8  dataTypeTo=int16  useOffsetTo=off  offsetToSrc=Specify via dialog  offsetTo=0  strideTo=1  sampleTime=inf  useInitValue=off  initValueSrc=Specify constant value  initValue=1  initValueSrcCode=myInitValueVariable  useAsMask=off  maskOperator=bitwise AND  useTermValue=off  termValue=1  isRealtimeEnabled=off  emitCCBeforeWrite=off  CCBeforeWrite=/* Custom Code Before Write*/  emitCCAfterWrite=off  CCAfterWrite=/* Custom Code After Write*/  useDMACopy=off  enableBlockingMode=off
  p1 : idelinklib_common/Memory Copy  copyFrom=Specified source code symbol  copyFromAddressSource=Specify via dialog  copyFromAddress=hex2dec('00200000')  copyFromSrcCode=p1  dataTypeFrom=int16  dataDimensionFrom=1  useOffsetFrom=off  offsetFromSrc=Specify via dialog  offsetFrom=0  strideFrom=1  copyTo=Output port  copyToAddressSource=Specify via dialog  copyToAddress=hex2dec('00002000')  copyToSrcCode=p1  dataTypeTo=int16  useOffsetTo=off  offsetToSrc=Specify via dialog  offsetTo=0  strideTo=1  sampleTime=inf  useInitValue=off  initValueSrc=Specify constant value  initValue=1  initValueSrcCode=myInitValueVariable  useAsMask=off  maskOperator=bitwise AND  useTermValue=off  termValue=1  isRealtimeEnabled=off  emitCCBeforeWrite=off  CCBeforeWrite=/* Custom Code Before Write*/  emitCCAfterWrite=off  CCAfterWrite=/* Custom Code After Write*/  useDMACopy=off  enableBlockingMode=off
  p2 : idelinklib_common/Memory Copy  copyFrom=Specified source code symbol  copyFromAddressSource=Specify via dialog  copyFromAddress=hex2dec('00200000')  copyFromSrcCode=p2  dataTypeFrom=int16  dataDimensionFrom=1  useOffsetFrom=off  offsetFromSrc=Specify via dialog  offsetFrom=0  strideFrom=1  copyTo=Output port  copyToAddressSource=Specify via dialog  copyToAddress=hex2dec('00002000')  copyToSrcCode=p1  dataTypeTo=int16  useOffsetTo=off  offsetToSrc=Specify via dialog  offsetTo=0  strideTo=1  sampleTime=inf  useInitValue=off  initValueSrc=Specify constant value  initValue=1  initValueSrcCode=myInitValueVariable  useAsMask=off  maskOperator=bitwise AND  useTermValue=off  termValue=1  isRealtimeEnabled=off  emitCCBeforeWrite=off  CCBeforeWrite=/* Custom Code Before Write*/  emitCCAfterWrite=off  CCAfterWrite=/* Custom Code After Write*/  useDMACopy=off  enableBlockingMode=off
  p3 : idelinklib_common/Memory Copy  copyFrom=Specified source code symbol  copyFromAddressSource=Specify via dialog  copyFromAddress=hex2dec('00200000')  copyFromSrcCode=p3  dataTypeFrom=int16  dataDimensionFrom=1  useOffsetFrom=off  offsetFromSrc=Specify via dialog  offsetFrom=0  strideFrom=1  copyTo=Output port  copyToAddressSource=Specify via dialog  copyToAddress=hex2dec('00002000')  copyToSrcCode=p1  dataTypeTo=int16  useOffsetTo=off  offsetToSrc=Specify via dialog  offsetTo=0  strideTo=1  sampleTime=inf  useInitValue=off  initValueSrc=Specify constant value  initValue=1  initValueSrcCode=myInitValueVariable  useAsMask=off  maskOperator=bitwise AND  useTermValue=off  termValue=1  isRealtimeEnabled=off  emitCCBeforeWrite=off  CCBeforeWrite=/* Custom Code Before Write*/  emitCCAfterWrite=off  CCAfterWrite=/* Custom Code After Write*/  useDMACopy=off  enableBlockingMode=off
  p5 : idelinklib_common/Memory Copy  copyFrom=Specified source code symbol  copyFromAddressSource=Specify via dialog  copyFromAddress=hex2dec('00200000')  copyFromSrcCode=p5  dataTypeFrom=int16  dataDimensionFrom=1  useOffsetFrom=off  offsetFromSrc=Specify via dialog  offsetFrom=0  strideFrom=1  copyTo=Output port  copyToAddressSource=Specify via dialog  copyToAddress=hex2dec('00002000')  copyToSrcCode=p1  dataTypeTo=int16  useOffsetTo=off  offsetToSrc=Specify via dialog  offsetTo=0  strideTo=1  sampleTime=inf  useInitValue=off  initValueSrc=Specify constant value  initValue=1  initValueSrcCode=myInitValueVariable  useAsMask=off  maskOperator=bitwise AND  useTermValue=off  termValue=1  isRealtimeEnabled=off  emitCCBeforeWrite=off  CCBeforeWrite=/* Custom Code Before Write*/  emitCCAfterWrite=off  CCAfterWrite=/* Custom Code After Write*/  useDMACopy=off  enableBlockingMode=off
  p6 : idelinklib_common/Memory Copy  copyFrom=Specified source code symbol  copyFromAddressSource=Specify via dialog  copyFromAddress=hex2dec('00200000')  copyFromSrcCode=p6  dataTypeFrom=int16  dataDimensionFrom=1  useOffsetFrom=off  offsetFromSrc=Specify via dialog  offsetFrom=0  strideFrom=1  copyTo=Output port  copyToAddressSource=Specify via dialog  copyToAddress=hex2dec('00002000')  copyToSrcCode=p1  dataTypeTo=int16  useOffsetTo=off  offsetToSrc=Specify via dialog  offsetTo=0  strideTo=1  sampleTime=inf  useInitValue=off  initValueSrc=Specify constant value  initValue=1  initValueSrcCode=myInitValueVariable  useAsMask=off  maskOperator=bitwise AND  useTermValue=off  termValue=1  isRealtimeEnabled=off  emitCCBeforeWrite=off  CCBeforeWrite=/* Custom Code Before Write*/  emitCCAfterWrite=off  CCAfterWrite=/* Custom Code After Write*/  useDMACopy=off  enableBlockingMode=off
  p7 : idelinklib_common/Memory Copy  copyFrom=Specified source code symbol  copyFromAddressSource=Specify via dialog  copyFromAddress=hex2dec('00200000')  copyFromSrcCode=p7  dataTypeFrom=int16  dataDimensionFrom=1  useOffsetFrom=off  offsetFromSrc=Specify via dialog  offsetFrom=0  strideFrom=1  copyTo=Output port  copyToAddressSource=Specify via dialog  copyToAddress=hex2dec('00002000')  copyToSrcCode=p1  dataTypeTo=int16  useOffsetTo=off  offsetToSrc=Specify via dialog  offsetTo=0  strideTo=1  sampleTime=inf  useInitValue=off  initValueSrc=Specify constant value  initValue=1  initValueSrcCode=myInitValueVariable  useAsMask=off  maskOperator=bitwise AND  useTermValue=off  termValue=1  isRealtimeEnabled=off  emitCCBeforeWrite=off  CCBeforeWrite=/* Custom Code Before Write*/  emitCCAfterWrite=off  CCAfterWrite=/* Custom Code After Write*/  useDMACopy=off  enableBlockingMode=off
  UD : Outport
  UOUT : Outport  Port=2
  UOUT1 : Outport  Port=3
  FREQ : Outport  Port=4
  IA : Outport  Port=5
  IB : Outport  Port=6
  wires:
  p1/1 -> UD/1
  p2/1 -> UOUT/1
  p3/1 -> UOUT1/1
  p5/1 -> FREQ/1
  p6/1 -> IA/1
  p7/1 -> IB/1

== system PMSM20180521/Subsystem1/PI-Nr/RC filter8 ==
  x : Inport
  Constant2 : Constant  Value=a  OutDataTypeStr=double
  Constant3 : Constant  Value=1-a  OutDataTypeStr=double
  Divide : Product
  Divide1 : Product
  Sum2 : Sum
  Unit Delay2 : UnitDelay  SampleTime=-1
  y : Outport
  wires:
  Unit Delay2/1 -> Divide1/2
  Sum2/1 -> Unit Delay2/1, y/1
  Divide1/1 -> Sum2/2
  Divide/1 -> Sum2/1
  Constant3/1 -> Divide1/1
  Constant2/1 -> Divide/2
  x/1 -> Divide/1

== system PMSM20180521/Subsystem1/SPWM/Clarke1 ==
  In1 : Inport
  In2 : Inport  Port=2
  Constant58 : Constant  Value=3  OutDataTypeStr=double
  Divide : Product  Inputs=*/
  Gain : Gain  Gain=2
  Gain1 : Gain
  Gain2 : Gain
  Sqrt : Sqrt  SaturateOnIntegerOverflow=on
  Sum : Sum
  alpha : Outport
  beta : Outport  Port=2
  wires:
  Divide/1 -> Gain2/1
  Sqrt/1 -> Divide/2
  Constant58/1 -> Sqrt/1
  Sum/1 -> Divide/1
  Gain/1 -> Sum/2
  In1/1 -> Sum/1, Gain1/1
  In2/1 -> Gain/1
  Gain1/1 -> alpha/1
  Gain2/1 -> beta/1

== system PMSM20180521/Subsystem1/abc/dq current/Clarke1 ==
  In1 : Inport
  In2 : Inport  Port=2
  Constant58 : Constant  Value=3  OutDataTypeStr=double
  Divide : Product  Inputs=*/
  Gain : Gain  Gain=2
  Sqrt : Sqrt  SaturateOnIntegerOverflow=on
  Sum : Sum
  alpha : Outport
  beta : Outport  Port=2
  wires:
  Divide/1 -> beta/1
  Sqrt/1 -> Divide/2
  Constant58/1 -> Sqrt/1
  Sum/1 -> Divide/1
  Gain/1 -> Sum/2
  In1/1 -> Sum/1, alpha/1
  In2/1 -> Gain/1

== system PMSM20180521/Subsystem1/abc/dq current/Park1 ==
  alpha : Inport
  beta : Inport  Port=2
  theta : Inport  Port=3
  Add4 : Sum
  Add5 : Sum
  Gain1 : Gain  Gain=-1
  Product{,1..3} (4 alike) : Product  RndMeth=Zero
  cos : Trigonometry  Operator=cos
  sin : Trigonometry
  d : Outport
  q : Outport  Port=2
  wires:
  Product3/1 -> Add5/2
  Gain1/1 -> Add5/1
  Product2/1 -> Gain1/1
  Product/1 -> Add4/2
  Product1/1 -> Add4/1
  alpha/1 -> Product1/1, Product2/2
  Add4/1 -> d/1
  theta/1 -> cos/1, sin/1
  Add5/1 -> q/1
  cos/1 -> Product1/2, Product3/1
  beta/1 -> Product/2, Product3/2
  sin/1 -> Product/1, Product2/1

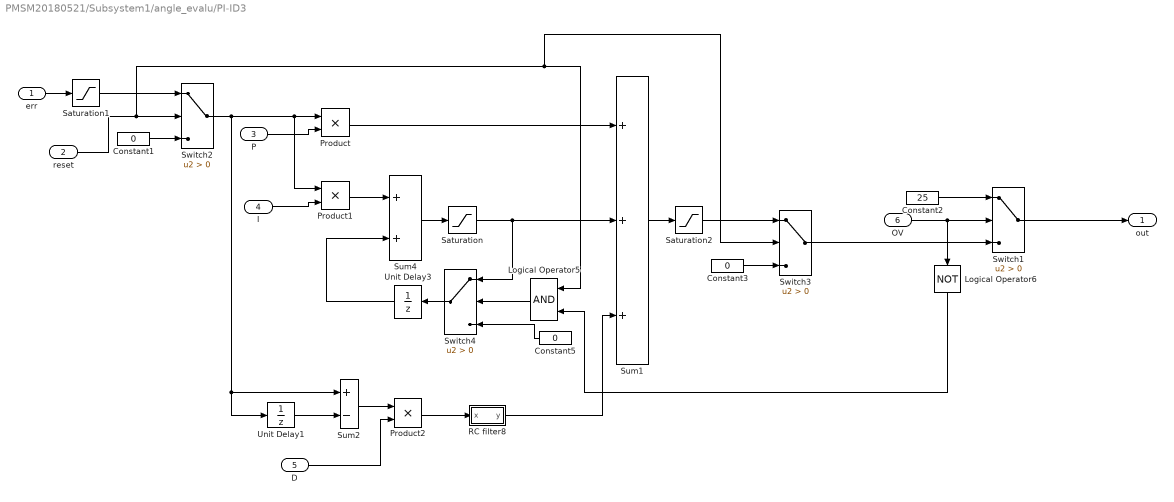
== system PMSM20180521/Subsystem1/angle_evalu/PI-ID3 ==
  err : Inport
  reset : Inport  Port=2
  P : Inport  Port=3
  I : Inport  Port=4
  D : Inport  Port=5
  OV : Inport  Port=6
  Constant1 : Constant  Value=0  OutDataTypeStr=Inherit: Inherit via back propagation
  Constant2 : Constant  Value=25  OutDataTypeStr=Inherit: Inherit via back propagation
  Constant3 : Constant  Value=0  OutDataTypeStr=Inherit: Inherit via back propagation
  Constant5 : Constant  Value=0  OutDataTypeStr=Inherit: Inherit via back propagation
  Logical Operator5 : Logic  AllPortsSameDT=off  OutDataTypeStr=boolean
  Logical Operator6 : Logic  Operator=NOT  AllPortsSameDT=off  OutDataTypeStr=boolean
  Product : Product  RndMeth=Zero
  Product1 : Product  RndMeth=Zero
  Product2 : Product  RndMeth=Zero
  RC filter8 : Subsystem  mask{a=0.4}
      mask prompts: a "Time Constant"
  Saturation : Saturate  UpperLimit=max  LowerLimit=min  LinearizeAsGain=off  ZeroCross=off  OutDataTypeStr=double
  Saturation1 : Saturate  UpperLimit=ermax  LowerLimit=ermin  LinearizeAsGain=off  ZeroCross=off  OutDataTypeStr=double
  Saturation2 : Saturate  UpperLimit=max  LowerLimit=min  LinearizeAsGain=off  ZeroCross=off  OutDataTypeStr=double
  Sum1 : Sum  Inputs=+++
  Sum2 : Sum  Inputs=+-
  Sum4 : Sum
  Switch{1..4} (4 alike) : Switch  Criteria=u2 > Threshold  SaturateOnIntegerOverflow=on  InputSameDT=on
  Unit Delay1 : UnitDelay  SampleTime=-1
  Unit Delay3 : UnitDelay  SampleTime=-1
  out : Outport
  wires:
  Logical Operator6/1 -> Logical Operator5/2
  Logical Operator5/1 -> Switch4/2
  RC filter8/1(y) -> Sum1/3
  Constant3/1 -> Switch3/3
  Switch3/1 -> Switch1/3
  Saturation2/1 -> Switch3/1
  Switch1/1 -> out/1
  OV/1 -> Logical Operator6/1, Switch1/2
  Constant2/1 -> Switch1/1
  Sum1/1 -> Saturation2/1
  Product2/1 -> RC filter8/1(x)
  Unit Delay1/1 -> Sum2/2
  D/1 -> Product2/2
  Sum2/1 -> Product2/1
  Switch4/1 -> Unit Delay3/1
  Unit Delay3/1 -> Sum4/2
  Saturation/1 -> Switch4/1, Sum1/2
  Sum4/1 -> Saturation/1
  Product1/1 -> Sum4/1
  I/1 -> Product1/2
  Product/1 -> Sum1/1
  Saturation1/1 -> Switch2/1
  err/1 -> Saturation1/1
  Constant1/1 -> Switch2/3
  reset/1 -> Logical Operator5/1, Switch3/2, Switch2/2
  Switch2/1 -> Unit Delay1/1, Sum2/1, Product1/1, Product/1
  P/1 -> Product/2
  Constant5/1 -> Switch4/3

== system PMSM20180521/Subsystem1/angle_evalu/RC filter3 ==
  x : Inport
  Constant2 : Constant  Value=a  OutDataTypeStr=double
  Constant3 : Constant  Value=1-a  OutDataTypeStr=double
  Divide : Product
  Divide1 : Product
  Sum2 : Sum
  Unit Delay2 : UnitDelay  SampleTime=-1
  y : Outport
  wires:
  Unit Delay2/1 -> Divide1/2
  Sum2/1 -> Unit Delay2/1, y/1
  Divide1/1 -> Sum2/2
  Divide/1 -> Sum2/1
  Constant3/1 -> Divide1/1
  Constant2/1 -> Divide/2
  x/1 -> Divide/1

== system PMSM20180521/Subsystem1/angle_evalu/angle generation ==
  freq : Inport
  Com : simulink/Logic and Bit Operations/Compare To Constant  relop=>=  const=2*pi  OutDataTypeStr=boolean
  Constant3 : Constant  Value=2*pi  OutDataTypeStr=double
  Rem : Math  Operator=rem  SaturateOnIntegerOverflow=on
  Sum11 : Sum
  Switch2 : Switch  Threshold=1
  Unit Delay1 : UnitDelay  SampleTime=-1
  angle_0 : Outport
  wires:
  Unit Delay1/1 -> Sum11/1
  freq/1 -> Sum11/2
  Sum11/1 -> Com/1, Switch2/3, Rem/1
  Switch2/1 -> angle_0/1, Unit Delay1/1
  Com/1 -> Switch2/2
  Rem/1 -> Switch2/1
  Constant3/1 -> Rem/2

== system PMSM20180521/Subsystem1/conversion/RC filter1 ==
  x : Inport
  Constant2 : Constant  Value=a  OutDataTypeStr=double
  Constant3 : Constant  Value=1-a  OutDataTypeStr=double
  Divide : Product
  Divide1 : Product
  Sum2 : Sum
  Unit Delay2 : UnitDelay  SampleTime=-1
  y : Outport
  wires:
  x/1 -> Divide/1
  Constant2/1 -> Divide/2
  Constant3/1 -> Divide1/1
  Divide/1 -> Sum2/1
  Divide1/1 -> Sum2/2
  Sum2/1 -> y/1, Unit Delay2/1
  Unit Delay2/1 -> Divide1/2

== system PMSM20180521/Subsystem1/conversion/RC filter2 ==
  x : Inport
  Constant2 : Constant  Value=a  OutDataTypeStr=double
  Constant3 : Constant  Value=1-a  OutDataTypeStr=double
  Divide : Product
  Divide1 : Product
  Sum2 : Sum
  Unit Delay2 : UnitDelay  SampleTime=-1
  y : Outport
  wires:
  Unit Delay2/1 -> Divide1/2
  Sum2/1 -> Unit Delay2/1, y/1
  Divide1/1 -> Sum2/2
  Divide/1 -> Sum2/1
  Constant3/1 -> Divide1/1
  Constant2/1 -> Divide/2
  x/1 -> Divide/1

== system PMSM20180521/Subsystem1/conversion/RC filter3 ==
  x : Inport
  Constant2 : Constant  Value=a  OutDataTypeStr=double
  Constant3 : Constant  Value=1-a  OutDataTypeStr=double
  Divide : Product
  Divide1 : Product
  Sum2 : Sum
  Unit Delay2 : UnitDelay  SampleTime=-1
  y : Outport
  wires:
  Unit Delay2/1 -> Divide1/2
  Sum2/1 -> Unit Delay2/1, y/1
  Divide1/1 -> Sum2/2
  Divide/1 -> Sum2/1
  Constant3/1 -> Divide1/1
  Constant2/1 -> Divide/2
  x/1 -> Divide/1

== system PMSM20180521/Subsystem1/conversion/RC filter4 ==
  x : Inport
  Constant2 : Constant  Value=a  OutDataTypeStr=double
  Constant3 : Constant  Value=1-a  OutDataTypeStr=double
  Divide : Product
  Divide1 : Product
  Sum2 : Sum
  Unit Delay2 : UnitDelay  SampleTime=-1
  y : Outport
  wires:
  Unit Delay2/1 -> Divide1/2
  Sum2/1 -> Unit Delay2/1, y/1
  Divide1/1 -> Sum2/2
  Divide/1 -> Sum2/1
  Constant3/1 -> Divide1/1
  Constant2/1 -> Divide/2
  x/1 -> Divide/1

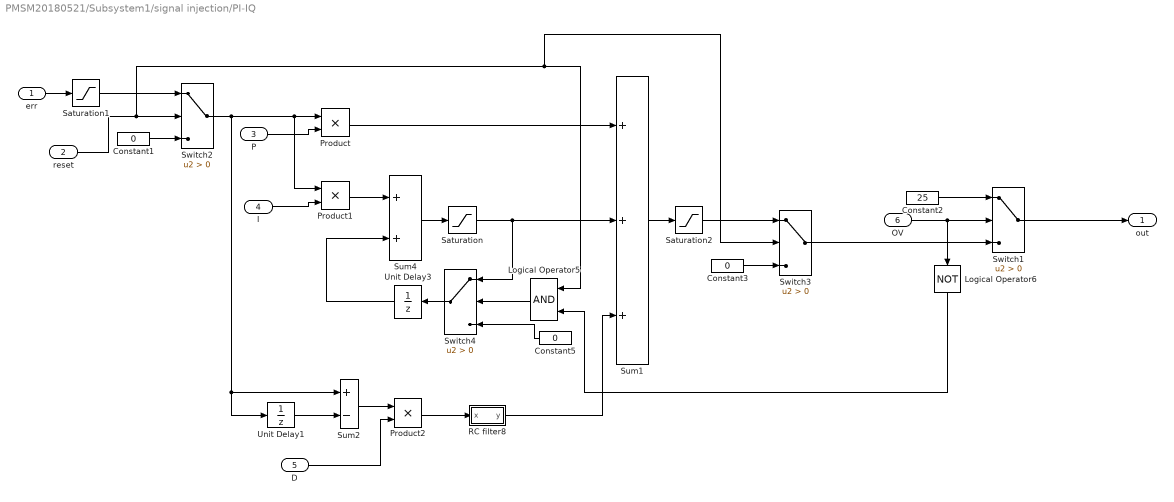
== system PMSM20180521/Subsystem1/signal injection/PI-IQ ==
  err : Inport
  reset : Inport  Port=2
  P : Inport  Port=3
  I : Inport  Port=4
  D : Inport  Port=5
  OV : Inport  Port=6
  Constant1 : Constant  Value=0  OutDataTypeStr=Inherit: Inherit via back propagation
  Constant2 : Constant  Value=25  OutDataTypeStr=Inherit: Inherit via back propagation
  Constant3 : Constant  Value=0  OutDataTypeStr=Inherit: Inherit via back propagation
  Constant5 : Constant  Value=0  OutDataTypeStr=Inherit: Inherit via back propagation
  Logical Operator5 : Logic  AllPortsSameDT=off  OutDataTypeStr=boolean
  Logical Operator6 : Logic  Operator=NOT  AllPortsSameDT=off  OutDataTypeStr=boolean
  Product : Product  RndMeth=Zero
  Product1 : Product  RndMeth=Zero
  Product2 : Product  RndMeth=Zero
  RC filter8 : Subsystem  mask{a=0.4}
      mask prompts: a "Time Constant"
  Saturation : Saturate  UpperLimit=max  LowerLimit=min  LinearizeAsGain=off  ZeroCross=off  OutDataTypeStr=double
  Saturation1 : Saturate  UpperLimit=ermax  LowerLimit=ermin  LinearizeAsGain=off  ZeroCross=off  OutDataTypeStr=double
  Saturation2 : Saturate  UpperLimit=max  LowerLimit=min  LinearizeAsGain=off  ZeroCross=off  OutDataTypeStr=double
  Sum1 : Sum  Inputs=+++
  Sum2 : Sum  Inputs=+-
  Sum4 : Sum
  Switch{1..4} (4 alike) : Switch  Criteria=u2 > Threshold  SaturateOnIntegerOverflow=on  InputSameDT=on
  Unit Delay1 : UnitDelay  SampleTime=-1
  Unit Delay3 : UnitDelay  SampleTime=-1
  out : Outport
  wires:
  Constant5/1 -> Switch4/3
  P/1 -> Product/2
  Switch2/1 -> Product/1, Product1/1, Sum2/1, Unit Delay1/1
  reset/1 -> Switch2/2, Switch3/2, Logical Operator5/1
  Constant1/1 -> Switch2/3
  err/1 -> Saturation1/1
  Saturation1/1 -> Switch2/1
  Product/1 -> Sum1/1
  I/1 -> Product1/2
  Product1/1 -> Sum4/1
  Sum4/1 -> Saturation/1
  Saturation/1 -> Sum1/2, Switch4/1
  Unit Delay3/1 -> Sum4/2
  Switch4/1 -> Unit Delay3/1
  Sum2/1 -> Product2/1
  D/1 -> Product2/2
  Unit Delay1/1 -> Sum2/2
  Product2/1 -> RC filter8/1(x)
  Sum1/1 -> Saturation2/1
  Constant2/1 -> Switch1/1
  OV/1 -> Switch1/2, Logical Operator6/1
  Switch1/1 -> out/1
  Saturation2/1 -> Switch3/1
  Switch3/1 -> Switch1/3
  Constant3/1 -> Switch3/3
  RC filter8/1(y) -> Sum1/3
  Logical Operator5/1 -> Switch4/2
  Logical Operator6/1 -> Logical Operator5/2

== system PMSM20180521/Subsystem1/signal injection/RC filter1 ==
  x : Inport
  Constant2 : Constant  Value=a  OutDataTypeStr=double
  Constant3 : Constant  Value=1-a  OutDataTypeStr=double
  Divide : Product
  Divide1 : Product
  Sum2 : Sum
  Unit Delay2 : UnitDelay  SampleTime=-1
  y : Outport
  wires:
  x/1 -> Divide/1
  Constant2/1 -> Divide/2
  Constant3/1 -> Divide1/1
  Divide/1 -> Sum2/1
  Divide1/1 -> Sum2/2
  Sum2/1 -> y/1, Unit Delay2/1
  Unit Delay2/1 -> Divide1/2

== system PMSM20180521/Subsystem1/signal injection/RC filter2 ==
  x : Inport
  Constant2 : Constant  Value=a  OutDataTypeStr=double
  Constant3 : Constant  Value=1-a  OutDataTypeStr=double
  Divide : Product
  Divide1 : Product
  Sum2 : Sum
  Unit Delay2 : UnitDelay  SampleTime=-1
  y : Outport
  wires:
  Unit Delay2/1 -> Divide1/2
  Sum2/1 -> Unit Delay2/1, y/1
  Divide1/1 -> Sum2/2
  Divide/1 -> Sum2/1
  Constant3/1 -> Divide1/1
  Constant2/1 -> Divide/2
  x/1 -> Divide/1

== system PMSM20180521/Subsystem1/signal injection/angle generation ==
  freq : Inport
  Com : simulink/Logic and Bit Operations/Compare To Constant  relop=>=  const=2*pi  OutDataTypeStr=boolean
  Constant3 : Constant  Value=2*pi  OutDataTypeStr=double
  Rem : Math  Operator=rem  SaturateOnIntegerOverflow=on
  Sum11 : Sum
  Switch2 : Switch  Threshold=1
  Unit Delay1 : UnitDelay  SampleTime=-1
  angle_0 : Outport
  wires:
  Unit Delay1/1 -> Sum11/1
  freq/1 -> Sum11/2
  Sum11/1 -> Com/1, Switch2/3, Rem/1
  Switch2/1 -> angle_0/1, Unit Delay1/1
  Com/1 -> Switch2/2
  Rem/1 -> Switch2/1
  Constant3/1 -> Rem/2

== system PMSM20180521/Subsystem1/w_evalu/RC filter4 ==
  x : Inport
  Constant2 : Constant  Value=a  OutDataTypeStr=double
  Constant3 : Constant  Value=1-a  OutDataTypeStr=double
  Divide : Product
  Divide1 : Product
  Sum2 : Sum
  Unit Delay2 : UnitDelay  SampleTime=-1
  y : Outport
  wires:
  x/1 -> Divide/1
  Constant2/1 -> Divide/2
  Constant3/1 -> Divide1/1
  Divide/1 -> Sum2/1
  Divide1/1 -> Sum2/2
  Sum2/1 -> y/1, Unit Delay2/1
  Unit Delay2/1 -> Divide1/2

== system PMSM20180521/Subsystem1/angle_evalu/PI-ID3/RC filter8 ==
  x : Inport
  Constant2 : Constant  Value=a  OutDataTypeStr=double
  Constant3 : Constant  Value=1-a  OutDataTypeStr=double
  Divide : Product
  Divide1 : Product
  Sum2 : Sum
  Unit Delay2 : UnitDelay  SampleTime=-1
  y : Outport
  wires:
  Unit Delay2/1 -> Divide1/2
  Sum2/1 -> Unit Delay2/1, y/1
  Divide1/1 -> Sum2/2
  Divide/1 -> Sum2/1
  Constant3/1 -> Divide1/1
  Constant2/1 -> Divide/2
  x/1 -> Divide/1
